simulink model "hosmo2_sim"  (R2021b)
settings: Solver=ode5  StartTime=0.0  StopTime=10.0  FixedStep=10^(-4)  RelTol=1e-3
settings Model: Creator=wkw  LastModifiedBy=wkw

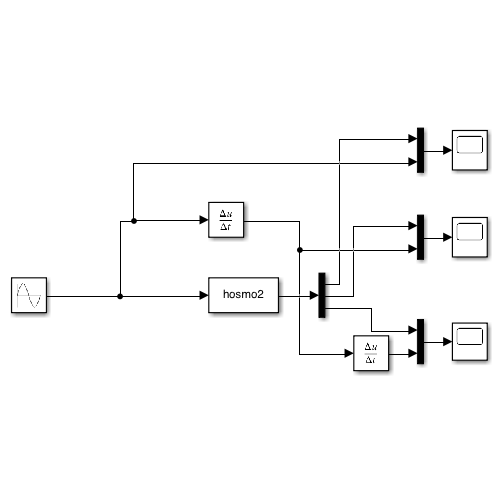
[thumbnail: Simulink's stored preview of the top-level diagram]
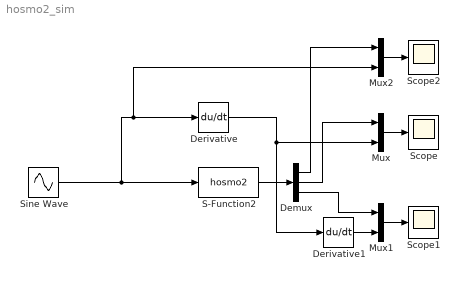
== system hosmo2_sim ==
  Demux : Demux  Outputs=3
  Derivative : Derivative
  Derivative1 : Derivative
  Mux : Mux  Inputs=2
  Mux1 : Mux  Inputs=2
  Mux2 : Mux  Inputs=2
  S-Function2 : S-Function  FunctionName=hosmo2  SFunctionDeploymentMode=off  EnableBusSupport=off
  Scope : Scope
  Scope1 : Scope
  Scope2 : Scope
  Sine Wave : Sin  SampleTime=0
  wires:
  Sine Wave/1 -> S-Function2/1, Mux2/2, Derivative/1
  S-Function2/1 -> Demux/1
  Mux1/1 -> Scope1/1
  Demux/3 -> Mux1/1
  Derivative/1 -> Derivative1/1, Mux/2
  Mux/1 -> Scope/1
  Demux/2 -> Mux/1
  Derivative1/1 -> Mux1/2
  Mux2/1 -> Scope2/1
  Demux/1 -> Mux2/1
